simulink model "fuzzy_pid"  (R2022b)
settings: Solver=VariableStepAuto  StartTime=0.0  StopTime=600  RelTol=1e-3
model workspace (MAT data in the model file):
  Kd = 0.01
  Ke = 1
  Kec = 1
  Ki = 0.01
  Kp = 0.1
  Ku = 0.05
  x_Kd = 0
  x_Ki = 0.03
  x_Kp = 0.02
undefined symbols (not defined in the file): DiscIntNeverNeededParam
libraries: simulink x3, fuzblock x1, slpidlib x1
settings Model: Creator=Lumos  LastModifiedBy=Lumos

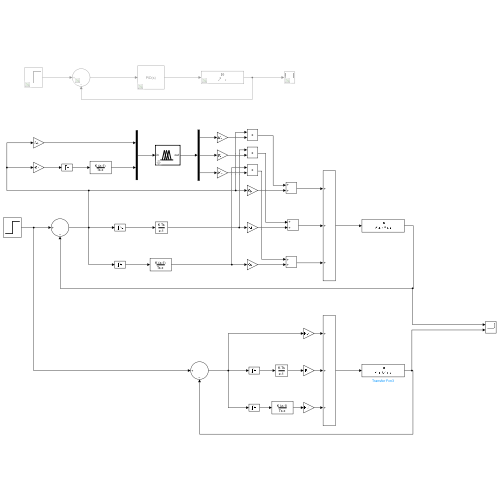
[thumbnail: Simulink's stored preview of the top-level diagram]
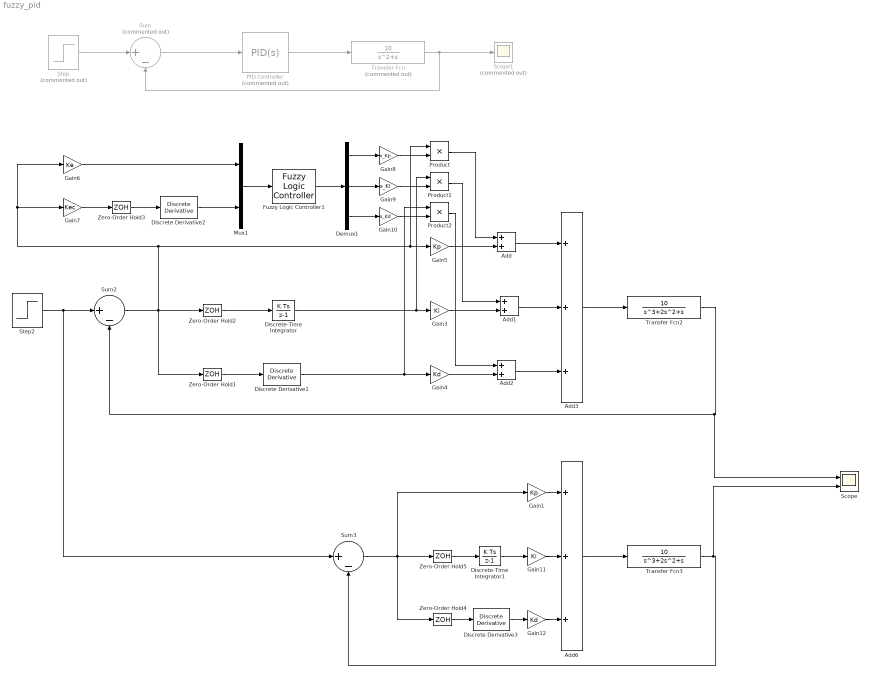
== system fuzzy_pid ==
  Add : Sum
  Add1 : Sum
  Add2 : Sum
  Add3 : Sum  Inputs=+++
  Add6 : Sum  Inputs=+++
  Demux1 : Demux  Outputs=3
  Discrete Derivative1 : simulink/Discrete/Discrete Derivative  gainval=1.0  ICPrevScaledInput=0.0  OutMin=[]  OutMax=[]  OutDataType=fixdt(1, 16)  OutScaling=2^-10  DoSatur=off
  Discrete Derivative2 : simulink/Discrete/Discrete Derivative  gainval=1.0  ICPrevScaledInput=0.0  OutMin=[]  OutMax=[]  OutDataType=fixdt(1, 16)  OutScaling=2^-10  DoSatur=off
  Discrete Derivative3 : simulink/Discrete/Discrete Derivative  gainval=1.0  ICPrevScaledInput=0.0  OutMin=[]  OutMax=[]  OutDataType=fixdt(1, 16)  OutScaling=2^-10  DoSatur=off
  Discrete-Time Integrator : DiscreteIntegrator  SampleTime=-1  ICPrevOutput=DiscIntNeverNeededParam  ICPrevScaledInput=DiscIntNeverNeededParam
  Discrete-Time Integrator1 : DiscreteIntegrator  SampleTime=-1  ICPrevOutput=DiscIntNeverNeededParam  ICPrevScaledInput=DiscIntNeverNeededParam
  Fuzzy Logic Controller1 : fuzblock/Fuzzy Logic  Controller  FIS=fuzzy_pid  OutputSampleNumber=101  DataType=double  FuzzifiedInputs=off  RuleFiringStrengths=off  RuleOutputs=off  AggregatedOutputs=off  SimulateUsing=Interpreted execution  OutOfRangeInputValueMessage=warning  NoRuleFiredMessage=warning  EmptyOutputFuzzySetMessage=warning
  Gain1 : Gain  Gain=Kp
  Gain10 : Gain  Gain=x_Kd
  Gain11 : Gain  Gain=Ki
  Gain12 : Gain  Gain=Kd
  Gain3 : Gain  Gain=Ki
  Gain4 : Gain  Gain=Kd
  Gain5 : Gain  Gain=Kp
  Gain6 : Gain  Gain=Ke
  Gain7 : Gain  Gain=Kec
  Gain8 : Gain  Gain=x_Kp
  Gain9 : Gain  Gain=x_Ki
  Mux1 : Mux  Inputs=2
  PID Controller : slpidlib/PID Controller  Commented=on  Controller=PID  Form=Parallel  TimeDomain=Continuous-time  UseExternalTs=off  SampleTime=-1  IntegratorMethod=Forward Euler  FilterMethod=Forward Euler  ControllerParametersSource=internal  P=0.5  I=0.2  UseKiTs=off  D=0.5  N=100  UseFilter=on  TunerSelectOption=Transfer Function Based (PID Tuner App)  InitialConditionSource=internal  InitialConditionForIntegrator=0  InitialConditionForFilter=0  DifferentiatorICPrevScaledInput=0  ExternalReset=none  TrackingMode=off  Kt=1  LimitOutput=off  SatLimitsSource=internal  UpperSaturationLimit=inf  LowerSaturationLimit=-inf  LinearizeAsGain=on  AntiWindupMode=none  Kb=1  LimitIntegrator=off  UpperIntegratorSaturationLimit=inf  LowerIntegratorSaturationLimit=-inf  POutMin=[]  POutMax=[]  IOutMin=[]  IOutMax=[]  DOutMin=[]  DOutMax=[]  NOutMin=[]  NOutMax=[]  SumOutMin=[]  SumOutMax=[]  SaturationOutMin=[]  SaturationOutMax=[]  PParamMin=[]  PParamMax=[]  IParamMin=[]  IParamMax=[]  DParamMin=[]  DParamMax=[]  NParamMin=[]  NParamMax=[]  KbParamMin=[]  KbParamMax=[]  KtParamMin=[]  KtParamMax=[]  KbOutMin=[]  KbOutMax=[]  KtOutMin=[]  KtOutMax=[]  IntegratorOutMin=[]  IntegratorOutMax=[]  FilterOutMin=[]  FilterOutMax=[]  SumI1OutMin=[]  SumI1OutMax=[]  SumI2OutMin=[]  SumI2OutMax=[]  SumI3OutMin=[]  SumI3OutMax=[]  SumI4OutMin=[]  SumI4OutMax=[]  SumDOutMin=[]  SumDOutMax=[]  DifferentiatorOutMin=[]  DifferentiatorOutMax=[]  FilterDiffOutCoefMin=[]  FilterDiffOutCoefMax=[]  ReciprocalOutMin=[]  ReciprocalOutMax=[]  SumDenOutMin=[]  SumDenOutMax=[]  SumNumOutMin=[]  SumNumOutMax=[]  DivideOutMin=[]  DivideOutMax=[]  UdiffTsProdOutMin=[]  UdiffTsProdOutMax=[]  NTsProdOutMin=[]  NTsProdOutMax=[]  UintegralTsProdOutMin=[]  UintegralTsProdOutMax=[]  UngainTsProdOutMin=[]  UngainTsProdOutMax=[]  ClampingZeroOutDataTypeStr=Inherit: Inherit via back propagation  ClampingZeroOutMin=[]  ClampingZeroOutMax=[]  FilterDenConstantOutDataTypeStr=Inherit: Inherit via back propagation  FilterDenConstantOutMin=[]  FilterDenConstantOutMax=[]  PCopyOutDataTypeStr=Inherit: Inherit via back propagation  PCopyOutMin=[]  PCopyOutMax=[]  NCopyOutDataTypeStr=Inherit: Inherit via back propagation  NCopyOutMin=[]  NCopyOutMax=[]  IntegratorContinuousStateAttributes=''  IntegratorStateMustResolveToSignalObject=off  IntegratorRTWStateStorageClass=Auto  FilterContinuousStateAttributes=''  FilterStateMustResolveToSignalObject=off  FilterRTWStateStorageClass=Auto  ParallelPVariant=InternalParameters  IdealPVariant=Disabled  IVariant=InternalParameters  DVariant=InternalParameters  IntegratorVariant=Continuous  SatVariant=Disabled  AWVariant=Passthrough  PCopyVariant=Disabled  TRVariant=Disabled  FdbkBlocksVariant=Forward  IdealPFdbkVariant=Disabled  SatFdbkVariant=Disabled  DerivativeFilterVariant=ContFilter  NVariant=InternalParameters  NCopyVariant=Disabled  FilterICVariant=InternalICsFilter  IntegratorICVariant=InternalICs  ExternalResetVariant=Disabled  TRSumVariant=Passthrough  SumFdbkVariant=Disabled  SumVariant=Sum_PID  TsampFilterVariant=InternalTs  TsampNgainVariant=Passthrough  TsampIntegralVariant=Passthrough  ExternalSaturationOutDataTypeStr=Inherit: Same as second input
  Product : Product
  Product1 : Product
  Product2 : Product
  Scope : Scope  NumInputPorts=2
  Scope1 : Scope  Commented=on
  Step : Step  Commented=on  SampleTime=0
  Step2 : Step  SampleTime=0
  Sum : Sum  Commented=on  Inputs=|+-
  Sum2 : Sum  Inputs=|+-
  Sum3 : Sum  Inputs=|+-
  Transfer Fcn : TransferFcn  Commented=on  Numerator=[10]  Denominator=[1 1 0]
  Transfer Fcn2 : TransferFcn  Numerator=[10]  Denominator=[1 2 1 0]
  Transfer Fcn3 : TransferFcn  Numerator=[10]  Denominator=[1 2 1 0]
  Zero-Order Hold{1..5} (5 alike) : ZeroOrderHold  SampleTime=-1
  wires:
  Step/1 -> Sum/1
  Transfer Fcn/1 -> Scope1/1, Sum/2
  Sum/1 -> PID Controller/1
  PID Controller/1 -> Transfer Fcn/1
  Step2/1 -> Sum3/1, Sum2/1
  Sum2/1 -> Gain6/1, Gain7/1, Product/1, Gain5/1, Zero-Order Hold1/1, Zero-Order Hold2/1
  Zero-Order Hold2/1 -> Discrete-Time Integrator/1
  Zero-Order Hold1/1 -> Discrete Derivative1/1
  Discrete-Time Integrator/1 -> Product1/1, Gain3/1
  Discrete Derivative1/1 -> Product2/1, Gain4/1
  Gain7/1 -> Zero-Order Hold3/1
  Zero-Order Hold3/1 -> Discrete Derivative2/1
  Gain6/1 -> Mux1/1
  Discrete Derivative2/1 -> Mux1/2
  Mux1/1 -> Fuzzy Logic Controller1/1
  Fuzzy Logic Controller1/1 -> Demux1/1
  Demux1/1 -> Gain8/1
  Demux1/2 -> Gain9/1
  Demux1/3 -> Gain10/1
  Gain8/1 -> Product/2
  Gain9/1 -> Product1/2
  Gain10/1 -> Product2/2
  Gain5/1 -> Add/2
  Product/1 -> Add/1
  Gain3/1 -> Add1/2
  Product1/1 -> Add1/1
  Gain4/1 -> Add2/2
  Product2/1 -> Add2/1
  Add/1 -> Add3/1
  Add1/1 -> Add3/2
  Add2/1 -> Add3/3
  Add3/1 -> Transfer Fcn2/1
  Transfer Fcn2/1 -> Scope/1, Sum2/2
  Transfer Fcn3/1 -> Scope/2, Sum3/2
  Zero-Order Hold4/1 -> Discrete Derivative3/1
  Add6/1 -> Transfer Fcn3/1
  Sum3/1 -> Gain1/1, Zero-Order Hold4/1, Zero-Order Hold5/1
  Discrete-Time Integrator1/1 -> Gain11/1
  Discrete Derivative3/1 -> Gain12/1
  Zero-Order Hold5/1 -> Discrete-Time Integrator1/1
  Gain11/1 -> Add6/2
  Gain12/1 -> Add6/3
  Gain1/1 -> Add6/1
